simulink model "wpt"  (R2021a)
settings: Solver=VariableStepAuto  StartTime=0.0  StopTime=10.0  RelTol=1e-3
libraries: spsSeriesRLCBranchLib x7, spsDiodeLib x5, spsCurrentMeasurementLib x4, spsIGBTDiodeLib x4, spsVoltageMeasurementLib x4, spsDCVoltageSourceLib x1, spsMosfetLib x1, spsMutualInductanceLib x1, spspowerguiLib x1
settings Model: Creator=Aditya  LastModifiedBy=Aditya

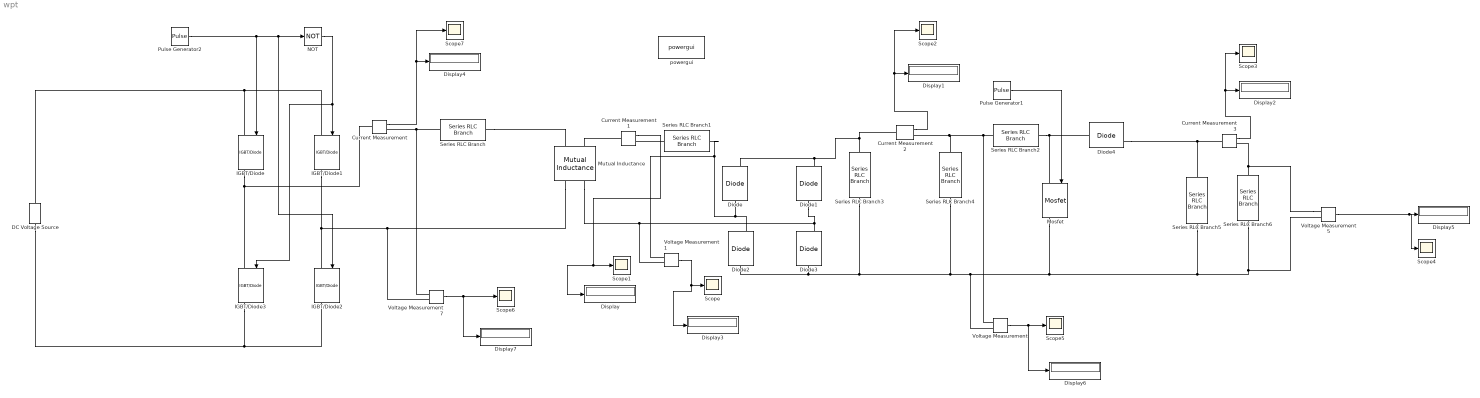
== system wpt ==
  Current Measurement{,1..3} (4 alike) : spsCurrentMeasurementLib/Current Measurement  PhasorSimulation=off  OutputType=Complex  PSBequivalent=0
  DC Voltage Source : spsDCVoltageSourceLib/DC Voltage Source  Amplitude=100  Measurements=None
  Diode{,1..4} (5 alike) : spsDiodeLib/Diode  Ron=0.001  Lon=0  Vf=0.8  IC=0  UseSnubber=0  Rs=500  Cs=250e-9  Measurements=on
  Display{,1..7} (8 alike) : Display
  IGBT/Diode{,1..3} (4 alike) : spsIGBTDiodeLib/IGBT//Diode  Ron=1e-3  Rs=1e5  Cs=inf  Measurements=on
  Mosfet : spsMosfetLib/Mosfet  Ron=0.001  Lon=0  Rd=0.001  Vfd=0  IC=0  Rs=1e5  Cs=inf  Measurements=on
  Mutual Inductance : spsMutualInductanceLib/Mutual Inductance  LConnTagsString=a|b  RConnTagsString=A|B  TypeOfMutual=Two or three windings with equal mutual terms  NumberOfWindings=3  SelfImpedance1=[.01 8.793e-05]  SelfImpedance2=[ .01 1.261e-04]  ThreeWindings=off  SelfImpedance3=[ 1.1 1.1e-03]  MutualImpedance=[0.1 2.106e-05]  InductanceMatrix="[1.0 0.9  0.9 ;  0.9 1.0  0.9;  0.9 0.9 1.0 ] * 1e-3"  ResistanceMatrix="[1.0 0.9  0.9 ;  0.9 1.0  0.9;  0.9 0.9 1.0 ]"  Measurements=None
      settings: SourceProductBaseCode=PS
  NOT : Logic  Operator=NOT  IconShape=distinctive  AllPortsSameDT=off  OutDataTypeStr=boolean
  Pulse Generator1 : DiscretePulseGenerator  PulseType=Time based  Period=1/25000  PulseWidth=70
  Pulse Generator2 : DiscretePulseGenerator  PulseType=Time based  Period=1/85000  PulseWidth=70
  Scope{,1..7} (8 alike) : Scope
  Series RLC Branch : spsSeriesRLCBranchLib/Series RLC Branch  LConnTagsString=__new0  RConnTagsString=__new0  BranchType=C  Resistance=1  Inductance=1e-3  SetiL0=off  InitialCurrent=0  Capacitance=4e-08  Setx0=off  InitialVoltage=0  Measurements=None
  Series RLC Branch1 : spsSeriesRLCBranchLib/Series RLC Branch  LConnTagsString=__new0  RConnTagsString=__new0  BranchType=C  Resistance=1  Inductance=1e-3  SetiL0=off  InitialCurrent=0  Capacitance=2.78e-08  Setx0=off  InitialVoltage=0  Measurements=None
  Series RLC Branch2 : spsSeriesRLCBranchLib/Series RLC Branch  LConnTagsString=__new0  RConnTagsString=__new0  BranchType=L  Resistance=1  Inductance=1e-3  SetiL0=off  InitialCurrent=0  Capacitance=1e-6  Setx0=off  InitialVoltage=0  Measurements=None
  Series RLC Branch3 : spsSeriesRLCBranchLib/Series RLC Branch  LConnTagsString=__new0  RConnTagsString=__new0  BranchType=C  Resistance=1  Inductance=1e-3  SetiL0=off  InitialCurrent=0  Capacitance=220e-06  Setx0=off  InitialVoltage=0  Measurements=None
  Series RLC Branch4 : spsSeriesRLCBranchLib/Series RLC Branch  LConnTagsString=__new0  RConnTagsString=__new0  BranchType=R  Resistance=100  Inductance=1e-3  SetiL0=off  InitialCurrent=0  Capacitance=1e-6  Setx0=off  InitialVoltage=0  Measurements=None
  Series RLC Branch5 : spsSeriesRLCBranchLib/Series RLC Branch  LConnTagsString=__new0  RConnTagsString=__new0  BranchType=C  Resistance=1  Inductance=1e-3  SetiL0=off  InitialCurrent=0  Capacitance=33e-06  Setx0=off  InitialVoltage=0  Measurements=None
  Series RLC Branch6 : spsSeriesRLCBranchLib/Series RLC Branch  LConnTagsString=__new0  RConnTagsString=__new0  BranchType=R  Resistance=100  Inductance=1e-3  SetiL0=off  InitialCurrent=0  Capacitance=1e-6  Setx0=off  InitialVoltage=0  Measurements=None
  Voltage Measurement{,1,5,7} (4 alike) : spsVoltageMeasurementLib/Voltage Measurement  PhasorSimulation=off  OutputType=Complex  PSBequivalent=0
  powergui : spspowerguiLib/powergui  Priority=1  SimulationMode=Discrete  SampleTime=1e-07  frequency=60  Iterations=50  frequencyindice=0  Pbase=100e6  ErrMax=1e-4  UnitsV=kV  UnitsW=MW  buscounter=0  FunctionMessages=off  echomessages=off  EnableUseOfTLC=off  CurrentSourceSwitches=off  DisableSnubberDevices=off  DisableRonSwitches=off  DisableVfSwitches=off  DisplayEquations=off  AutomaticDiscreteSolvers=off  SolverType=Tustin/Backward Euler (TBE)  Interpol=off  ExternalGateDelay=off  methode=off  Ts=100  x0status=blocks  SPID=on  SwTol=0  HookPort=off  NonlinearTolerance=1e-4  nMaxIteration=100  ContinueOnMaxIteration=off  RestoreLinks=warning  ResistiveCurrentMeasurement=off  Frange=[0:2:500]  Ylog=off  Xlog=on  ShowGrid=off  save=off  variable=ZData  structure=0  ZoomFFT=off  StartTime=0.0  cycles=1  DisplayStyle=1  fundamental=60  FreqAxis=off  MaxFrequency=1000  frequencyindicesteady=1  RmsSteady=1  display=off
  wires:
  Voltage Measurement1/1 -> Display3/1, Scope/1
  Current Measurement1/1 -> Display/1, Scope1/1
  Current Measurement2/1 -> Scope2/1, Display1/1
  Pulse Generator1/1 -> Mosfet/1
  Current Measurement3/1 -> Scope3/1, Display2/1
  Voltage Measurement5/1 -> Scope4/1, Display5/1
  Voltage Measurement/1 -> Display6/1, Scope5/1
  NOT/1 -> IGBT/Diode3/1, IGBT/Diode1/1
  Pulse Generator2/1 -> IGBT/Diode/1, IGBT/Diode2/1, NOT/1
  Current Measurement/1 -> Scope7/1, Display4/1
  Voltage Measurement7/1 -> Display7/1, Scope6/1
  connections:
  Mutual Inductance/RConn2 -- Current Measurement1/LConn1
  Series RLC Branch1/LConn1 -- Current Measurement1/RConn1
  Diode2/RConn1 -- Voltage Measurement1/LConn1 -- Series RLC Branch1/RConn1 -- Diode/LConn1
  Diode3/LConn1 -- Voltage Measurement/LConn2 -- Voltage Measurement5/LConn2 -- Series RLC Branch6/LConn1 -- Series RLC Branch5/RConn1 -- Mosfet/RConn1 -- Series RLC Branch4/LConn1 -- Series RLC Branch3/RConn1 -- Diode2/LConn1
  Diode1/LConn1 -- Voltage Measurement1/LConn2 -- Mutual Inductance/LConn2 -- Diode3/RConn1
  Diode1/RConn1 -- Current Measurement2/LConn1 -- Series RLC Branch3/LConn1 -- Diode/RConn1
  Voltage Measurement/LConn1 -- Series RLC Branch2/LConn1 -- Series RLC Branch4/RConn1 -- Current Measurement2/RConn1
  Series RLC Branch2/RConn1 -- Diode4/LConn1 -- Mosfet/LConn1
  Diode4/RConn1 -- Series RLC Branch5/LConn1 -- Current Measurement3/LConn1
  Voltage Measurement5/LConn1 -- Series RLC Branch6/RConn1 -- Current Measurement3/RConn1
  DC Voltage Source/RConn1 -- IGBT/Diode/LConn1 -- IGBT/Diode1/LConn1
  DC Voltage Source/LConn1 -- IGBT/Diode3/RConn1 -- IGBT/Diode2/RConn1
  IGBT/Diode/RConn1 -- Current Measurement/LConn1 -- IGBT/Diode3/LConn1
  IGBT/Diode1/RConn1 -- Voltage Measurement7/LConn2 -- Mutual Inductance/LConn1 -- IGBT/Diode2/LConn1
  Series RLC Branch/RConn1 -- Mutual Inductance/RConn1
  Voltage Measurement7/LConn1 -- Current Measurement/RConn1 -- Series RLC Branch/LConn1
